simulink model "TCMSSystem"  (R2019b)
settings: configuration reference "ConfigSet_TCMSSystem_Reference" (kept outside this file)
model workspace (MAT data in the model file):
  Prm_TCMSSystem : Simulink.Parameter (value not decoded)
  SampleTime = 0.05
symbols that are objects in the model workspace (value not decoded): Prm_TCMSSystem
undefined symbols (not defined in the file): ADDIntervention, AK1Status, AK2Status, AKContactorStatus, AllDoorsClosed, AllLeftDoorsClosed, AllRightDoorsClosed, APS1Fault, APS1Isolated, APS1OutputVoltage, APS1Status, APS2Fault, APS2Isolated, APS2OutputVoltage, APS2Status, APSKAKContactor, ASCOEnd1, ASCOEnd2, ATBMode, ATCBypassMode, ATCStatusNotOK, ATOMode, ATPLowSpeedCutoutStatus, ATPMode, AuxCompressor, BatteryCurrent, BatteryIsolationContactor, BatteryTemperature, BatteryVoltage, BCG1Fault, BCG1Isolated, BCG1IsolationFailed, BCG1OutputCurrent, BCG1Status, BCG2Fault, BCG2Isolated, BCG2OutputCurrent, BCG2Status, BCGOutputVoltage, BECU1AxleLockedWheelSet1, BECU2AxleLockedWheelSet2, BECUFaulty, BECUMajorFault, BECUMinorFault, BECUStatus, BIC1Inside, BIC1Outside, BIC2Inside, BIC2Outside, Bogie, Bogie1WSPStatus, Bogie2WSPStatus, BogieFaulty, BogieIsolationStatus, BogieSupportedMass, BrakeCylinderPressureGauge, BrakeLoopCBTripped, BrakeLoopOpenTL, BrakeTrainLineStatus, BrakingDemand ... (+215)
libraries: TimersLib x257, simulink x137, LatchesLib x42, VectorOperationsLib x15, TestBenchLib x12, MathOperationsLib x2, FiltersLib x1
(part 12 of 16)

== system TCMSSystem/TCMSSystemPerVehicle/EnabledTCMSVehicle/TCMSTractionBraking/TractionBrakingControl/CabControlsExtract/CabActiveTrainControl ==
  In Bus Element6 : Inport  PortName=DisplayControl  Element=EnableTractionPowerLimit
  In Bus Element5 : Inport  PortName=DisplayControl  Element=EDBrakingPowerLimit
  In Bus Element7 : Inport  PortName=DisplayControl  Element=EnableEDBrakingPowerLimit
  In Bus Element8 : Inport  PortName=DisplayControl  Element=MaxTractionAccelerationTargetOverride
  In Bus Element : Inport  PortName=DisplayControl  Element=MaxBrakingDecelerationTargetOverride
  In Bus Element1 : Inport  PortName=DisplayControl  Element=EnableTractionTargetOverride
  In Bus Element2 : Inport  PortName=DisplayControl  Element=EnableBrakingTargetOverride
  In Bus Element4 : Inport  PortName=DisplayControl  Element=TractionPowerLimit
  TractionCommand : Inport  Port=2
  BrakingCommand : Inport  Port=3
  HoldingBrakeStatus : Inport  Port=4
  TCMSSpeedLimit : Inport  Port=5
  LimitActive : Inport  Port=6
  HTERequired : Inport  Port=7
  WashModeActive : Inport  Port=8
  ShuntModeActive : Inport  Port=9
  ATPLowSpeedCutoutModeActive : Inport  Port=10
  Action Port : ActionPort  ActionPortLabel=if(u1 > 0)
  Bus Creator : BusCreator  Inputs=19  OutDataTypeStr=Bus: BD_TCMSSystem_Wires_TBTrainWire  NonVirtualBus=on
  Constant : Constant  Value=0
  Constant1 : Constant  Value=0
  Out1 : Outport
  wires:
  Bus Creator/1 -> Out1/1
  In Bus Element4/1 -> Bus Creator/1  "TractionPowerLimit"
  In Bus Element5/1 -> Bus Creator/2  "EDBrakingPowerLimit"
  In Bus Element6/1 -> Bus Creator/3  "EnableTractionPowerLimit"
  In Bus Element8/1 -> Bus Creator/5  "MaxTractionAccelerationTargetOverride"
  In Bus Element7/1 -> Bus Creator/4  "EnableEDBrakingPowerLimit"
  In Bus Element/1 -> Bus Creator/6  "MaxBrakingDecelerationTargetOverride"
  In Bus Element1/1 -> Bus Creator/7  "EnableTractionTargetOverride"
  In Bus Element2/1 -> Bus Creator/8  "EnableBrakingTargetOverride"
  BrakingCommand/1 -> Bus Creator/10  "BrakingCommand"
  TractionCommand/1 -> Bus Creator/9  "TractionCommand"
  HoldingBrakeStatus/1 -> Bus Creator/11  "HoldingBrakeStatus"
  TCMSSpeedLimit/1 -> Bus Creator/12  "TCMSSpeedLimit"
  LimitActive/1 -> Bus Creator/13  "Overspeed"
  Constant/1 -> Bus Creator/14  "EstimatedMass"
  HTERequired/1 -> Bus Creator/15  "HTERequired"
  WashModeActive/1 -> Bus Creator/16  "WashModeActive"
  Constant1/1 -> Bus Creator/17  "TractionForce"
  ShuntModeActive/1 -> Bus Creator/18  "ShuntModeActive"
  ATPLowSpeedCutoutModeActive/1 -> Bus Creator/19  "ATPLowSpeedCutoutModeActive"

== system TCMSSystem/TCMSSystemPerVehicle/EnabledTCMSVehicle/TCMSTractionBraking/TractionBrakingControl/CabControlsExtract/CabInactiveNoTrainControl ==
  Action Port : ActionPort  ActionPortLabel=else
  Constant3 : Constant  Value=0  OutDataTypeStr=Bus: BD_TCMSSystem_Wires_TBTrainWire
  Out1 : Outport
  wires:
  Constant3/1 -> Out1/1

== system TCMSSystem/TCMSSystemPerVehicle/EnabledTCMSVehicle/TCMSTractionBraking/TractionBrakingControl/CabControlsExtract/Speed Limit Protection ==
  ElectricalIn : Inport
  CBTCIn : Inport  Port=2
  IOControls : Inport  Port=3
  In Bus Element7 : Inport  Port=4  PortName=DisplayControl
  In Bus Element : Inport  Port=4  PortName=DisplayControl  Element=ActivateWashing3Kmph
  In Bus Element1 : Inport  Port=4  PortName=DisplayControl  Element=ActivateWashing4Kmph
  In Bus Element2 : Inport  Port=4  PortName=DisplayControl  Element=ActivateWashing5Kmph
  In Bus Element3 : Inport  Port=4  PortName=DisplayControl  Element=ShuntModeMaxSpeed
  In Bus Element4 : Inport  Port=4  PortName=DisplayControl  Element=ATPLowModeMaxSpeed
  In Bus Element5 : Inport  Port=4  PortName=DisplayControl  Element=ATPLowModeActivated
  In Bus Element6 : Inport  Port=4  PortName=DisplayControl  Element=ShuntModeActivated
  PneumaticsSystem : Inport  Port=5
  PneumaticsTrainSum : Inport  Port=6
  TractionBrakingBogieData : Inport  Port=7
  0kphConditions : Subsystem
  10kphConditions : Subsystem
  25kphConditions : Subsystem
  40kphConditions : Subsystem
  45kphConditions : Subsystem
  50kphConditions : Subsystem
  Bus Selector : BusSelector  OutputSignals=Speedometer
  Bus Selector2 : BusSelector  OutputSignals=Bogie
  Constant : Constant  Value=0
  Constant1 : Constant  Value=40
  Constant2 : Constant  Value=25
  Constant3 : Constant  Value=45
  Constant4 : Constant  Value=50
  Constant5 : Constant  Value=10
  Constant6 : Constant  Value=3
  Constant7 : Constant  Value=4
  Constant8 : Constant  Value=5
  OR : Logic  Operator=OR  Inputs=3  AllPortsSameDT=off  OutDataTypeStr=boolean
  SetByATCLimits : Constant  Value=0
  Special Modes Case : Subsystem
  Switch{,1..10} (11 alike) : Switch  Criteria=u2 > Threshold
  kphTomps{1..11} (11 alike) : Gain  Gain=1/3.6
  SpecialModesOverspeed : Outport
  TCMSSpeedLimit : Outport  Port=2
  LimitActive : Outport  Port=3
  WashModeActive : Outport  Port=4
  wires:
  Constant/1 -> Switch/1
  Constant2/1 -> kphTomps1/1
  kphTomps1/1 -> Switch2/1
  0kphConditions/1(True) -> Special Modes Case/7(SpeedRestrict), Switch/2  "6 or more bogies isolated"
  25kphConditions/1(True) -> Switch2/2  "LimpHome or Forward Mode"
  ElectricalIn/1 -> 40kphConditions/1(ElectricalIn), 25kphConditions/3(ElectricalIn), Bus Selector/1
  Switch2/1 -> Switch5/3
  CBTCIn/1 -> 10kphConditions/2(CBTCIn), 0kphConditions/3(CBTCIn), Special Modes Case/1(CBTCIn), 25kphConditions/2(CBTCIn)
  Bus Selector/1 -> Special Modes Case/3(<Speedometer>)  "<Speedometer>"
  40kphConditions/1(True) -> Switch1/2  "4 or more bogies isolated"
  kphTomps2/1 -> Switch10/3
  SetByATCLimits/1 -> kphTomps2/1
  Switch1/1 -> Switch2/3
  Constant1/1 -> kphTomps3/1
  45kphConditions/1(True) -> Switch3/2  "3 or more bogies isolated"
  Switch3/1 -> Switch1/3
  Constant3/1 -> kphTomps4/1
  50kphConditions/1(True) -> Switch4/2  "2 or more bogies isolated"
  Switch4/1 -> Switch3/3
  Constant4/1 -> kphTomps5/1
  kphTomps3/1 -> Switch1/1
  kphTomps4/1 -> Switch3/1
  kphTomps5/1 -> Switch4/1
  10kphConditions/1(True) -> Switch5/2  "Reverse mode"
  Switch5/1 -> Switch6/3
  Constant5/1 -> kphTomps6/1
  kphTomps6/1 -> Switch5/1
  Switch/1 -> Special Modes Case/4(SpeedLimit), TCMSSpeedLimit/1
  PneumaticsTrainSum/1 -> 45kphConditions/1(PneumaticTrainSum), 10kphConditions/1(PneumaticsIn), 0kphConditions/1(PneumaticTrainSum), 40kphConditions/2(PneumaticTrainSum), 50kphConditions/2(PneumaticTrainSum)
  TractionBrakingBogieData/1 -> 50kphConditions/3(TractionBrakingBogieData), 40kphConditions/3(TractionBrakingBogieData)
  Switch7/1 -> Switch/3
  Switch8/1 -> Switch7/3
  Switch6/1 -> Switch8/3
  In Bus Element/1 -> OR/1, Switch7/2
  In Bus Element1/1 -> OR/2, Switch8/2
  In Bus Element2/1 -> OR/3, Switch6/2
  kphTomps7/1 -> Switch7/1
  Constant6/1 -> kphTomps7/1
  Constant7/1 -> kphTomps8/1
  kphTomps8/1 -> Switch8/1
  kphTomps9/1 -> Switch6/1
  Constant8/1 -> kphTomps9/1
  PneumaticsSystem/1 -> Bus Selector2/1
  Bus Selector2/1 -> 40kphConditions/4(<Bogie>), 50kphConditions/1(<Bogie>)  "<Bogie>"
  OR/1 -> WashModeActive/1, Special Modes Case/2(WashModeActive)  "WashModeActive"
  IOControls/1 -> 0kphConditions/2(IOControls), Special Modes Case/5(IOControls), 25kphConditions/1(IOControls), 10kphConditions/3(IOControls)
  Special Modes Case/1(SpecialModesOverspeed) -> SpecialModesOverspeed/1
  Special Modes Case/2(SpecialLimitActive) -> LimitActive/1
  Switch9/1 -> Switch4/3
  kphTomps10/1 -> Switch9/1
  In Bus Element3/1 -> kphTomps10/1
  Switch10/1 -> Switch9/3
  In Bus Element6/1 -> Switch9/2
  In Bus Element4/1 -> kphTomps11/1
  In Bus Element5/1 -> Switch10/2
  In Bus Element7/1 -> Special Modes Case/6(DisplayControl)
  kphTomps11/1 -> Switch10/1

== system TCMSSystem/TCMSSystemPerVehicle/EnabledTCMSVehicle/TCMSTractionBraking/TractionBrakingControl/CabControlsExtract/TractionBrakingRefCalc ==
  note: In wash mode, for example, for 3KMPH set point, traction will be cut at 3 kmph,
      | 50% FSB shall be applied at 4 KMPH, and FSB shall be applied at 5 KMPH.
      | This logic is extended for 4 and 5 KMPH set points.
  note: TractionCutoutFault
  DynamicsIn : Inport
  CBTCSignals : Inport  Port=2
  InputState : Inport  Port=3
  TractionCmd : Inport  Port=4
  In Bus Element26 : Inport  Port=5  PortName=Faults  Element=BECUPWRAndBRKCmdAtSameTime
  In Bus Element : Inport  Port=5  PortName=Faults  Element=TractionCutModeSelectorInATPATOUTO
  SpecialModesOverspeed : Inport  Port=6
  Abs : Abs
  Bus Selector : BusSelector  OutputSignals=TractionBrakeController,ModeSelector
  Bus Selector1 : BusSelector  OutputSignals=VehicleSpeed
  Bus Selector2 : BusSelector  OutputSignals=BrakingCommand,TractionForce
  Bus Selector4 : BusSelector  OutputSignals=HoldingBrakeStatus
  Compare To Constant : simulink/Logic and Bit Operations/Compare To Constant  relop===  const=0  OutDataTypeStr=boolean
  Compare To Constant1 : simulink/Logic and Bit Operations/Compare To Constant  relop===  const=4  OutDataTypeStr=boolean
  Compare To Constant2 : simulink/Logic and Bit Operations/Compare To Constant  relop===  const=5  OutDataTypeStr=boolean
  Compare To Constant4 : simulink/Logic and Bit Operations/Compare To Constant  relop===  const=1  OutDataTypeStr=boolean
  Compare To Constant5 : simulink/Logic and Bit Operations/Compare To Constant  relop===  const=2  OutDataTypeStr=boolean
  Constant : Constant  Value=0
  Constant1 : Constant  Value=100
  Constant2 : Constant  Value=0
  Constant3 : Constant  Value=50
  Constant4 : Constant  Value=100
  Detect Increase : simulink/Logic and Bit Operations/Detect Increase  vinit=0.0  OutDataTypeStr=boolean
  Detect Increase1 : simulink/Logic and Bit Operations/Detect Increase  vinit=0.0  OutDataTypeStr=boolean
  HBRelease : Subsystem
  HoldingBrake : Subsystem
  Logical Operator : Logic  Operator=OR  Inputs=3  AllPortsSameDT=off  OutDataTypeStr=boolean
  Logical Operator1 : Logic  Operator=OR  AllPortsSameDT=off  OutDataTypeStr=boolean
  Logical Operator2 : Logic  Operator=OR  AllPortsSameDT=off  OutDataTypeStr=boolean
  Logical Operator3 : Logic  AllPortsSameDT=off  OutDataTypeStr=boolean
  Max : MinMax  Function=max  Inputs=2
  SR Latch - Reset Priority : LatchesLib/SR Latch - Reset Priority  initial_condition=0
      settings: SourceProductName=Latches
  Saturation : Saturate  UpperLimit=120  LowerLimit=0
  Saturation1 : Saturate  UpperLimit=0  LowerLimit=-120
  Switch{,1..6} (7 alike) : Switch  Criteria=u2 > Threshold
  TBRefDemandFromCBTC : Subsystem
  TractionCommand : Outport
  BrakingCommand : Outport  Port=2
  HoldingBrakesStatus : Outport  Port=3
  wires:
  TBRefDemandFromCBTC/1(ATO/UTOModeActive) -> [ATOMode], Switch2/2, Switch1/2
  CBTCSignals/1 -> TBRefDemandFromCBTC/1(CBTC)
  TBRefDemandFromCBTC/2(RefTraction) -> Switch1/1
  Switch5/1 -> BrakingCommand/1
  InputState/1 -> Bus Selector/1
  TBRefDemandFromCBTC/3(RefBraking) -> Switch2/1
  Saturation/1 -> Switch1/3  "TractionCommand"
  Bus Selector/1 -> Saturation1/1, Saturation/1  "<TractionBrakeController>"
  Saturation1/1 -> Abs/1
  Abs/1 -> Switch2/3  "BrakingCommand"
  HoldingBrake/1(HoldingBrakeDemand) -> Max/2
  HoldingBrake/2(HoldingBrakeApplied) -> HoldingBrakesStatus/1  "HoldingBrakeApplied"
  DynamicsIn/1 -> Bus Selector1/1
  Bus Selector1/1 -> HoldingBrake/2(VehicleSpeed)  "<VehicleSpeed>"
  HBRelease/1(HBRelease) -> HoldingBrake/3(TCMSHoldingBrakeRelease)
  [NotImmobilise] -> HBRelease/2(NotImmobilise)
  [ATOMode] -> HBRelease/3(ATO/UTO)
  TBRefDemandFromCBTC/5(NotImmobilise) -> [NotImmobilise]
  TBRefDemandFromCBTC/4(NoSB) -> Switch3/2, Switch/2
  Switch2/1 -> Switch3/1
  Switch1/1 -> Switch/1
  Switch4/1 -> TractionCommand/1
  Constant1/1 -> Switch3/3
  Constant/1 -> Switch/3
  TractionCmd/1 -> Bus Selector4/1, Bus Selector2/1
  Switch3/1 -> Max/1
  Bus Selector4/1 -> HBRelease/4(HBStatus)  "<HoldingBrakeStatus>"
  Switch/1 -> Switch4/3
  Bus Selector/2 -> [ModeSelector]  "<ModeSelector>"
  [ModeSelector] -> Compare To Constant2/1, Compare To Constant1/1, Compare To Constant/1
  Compare To Constant/1 -> Detect Increase1/1, Logical Operator/1
  Compare To Constant1/1 -> Logical Operator/2
  Compare To Constant2/1 -> Logical Operator/3
  Logical Operator/1 -> Logical Operator3/1
  Constant2/1 -> Switch4/1
  In Bus Element/1 -> Logical Operator3/2
  Logical Operator1/1 -> Switch4/2
  In Bus Element26/1 -> Detect Increase/1
  Detect Increase/1 -> SR Latch - Reset Priority/1
  Constant4/1 -> Switch5/1
  Logical Operator3/1 -> Logical Operator1/2
  Detect Increase1/1 -> SR Latch - Reset Priority/2
  Max/1 -> Switch6/3
  SpecialModesOverspeed/1 -> Compare To Constant5/1, Compare To Constant4/1
  SR Latch - Reset Priority/1 -> Logical Operator2/1, Logical Operator1/1
  Compare To Constant4/1 -> Logical Operator2/2
  Logical Operator2/1 -> Switch5/2
  Compare To Constant5/1 -> Switch6/2
  Constant3/1 -> Switch6/1
  Switch6/1 -> Switch5/3
  Bus Selector2/2 -> HBRelease/1(TractionForceFB)  "<TractionForce>"
  Bus Selector2/1 -> HoldingBrake/1(BrakingCommand)  "<BrakingCommand>"

== system TCMSSystem/TCMSSystemPerVehicle/EnabledTCMSVehicle/TCMSTractionBraking/TractionBrakingControl/ForEachBogie/Subsystem ==
  note: Brake blending, EP compensates what ED cannot provide
  note: SH: This update was done in Nov24 because the brake icon on brake screen should not
      | glow for T car until the speed is less than 7 KMPH.
      | Total brake demand is calculated per unit, hence it is important to compare it with
      | the ED brake achieved per unit in order to calculate the EP demand (deficit). But at lower speed
      | when ED efforts are fading out, the brake demand is compared per vehicle and T cars are the first one to get the EP demand,
      | until there is still some ED brake efforts possible in DM/M cars.
      | This also improves the max and avg acceleration (ED+EP).
  EffortsAchievedPerUnit : Inport
  Speed : Inport  Port=2
  EffortsAchivedPerVehicle : Inport  Port=3
  Abs : Abs
  Bus Selector2 : BusSelector  OutputSignals=EDBrakingEffortAchieved
  Bus Selector3 : BusSelector  OutputSignals=EDBrakingEffortAchieved
  Bus Selector4 : BusSelector  OutputSignals=VehicleSpeed
  Switch1 : Switch  Criteria=u2 > Threshold  Threshold=1.75
  SelectEPBrakeDemand : Outport
  wires:
  Bus Selector3/1 -> Switch1/1  "<EDBrakingEffortAchieved>"
  Switch1/1 -> SelectEPBrakeDemand/1
  Bus Selector2/1 -> Switch1/3  "<EDBrakingEffortAchieved>"
  EffortsAchivedPerVehicle/1 -> Bus Selector2/1
  Bus Selector4/1 -> Abs/1  "<VehicleSpeed>"
  Abs/1 -> Switch1/2
  EffortsAchievedPerUnit/1 -> Bus Selector3/1
  Speed/1 -> Bus Selector4/1

== system TCMSSystem/TCMSSystemPerVehicle/EnabledTCMSVehicle/TCMSTractionBraking/TractionBrakingDisplay/BrakeScreen/For Each Subsystem ==
  In1 : Inport  Partition=on  PartitionDimension=1  PartitionWidth=1  PartitionOffset=0
  Bus Selector : BusSelector  OutputSignals=TCUSlideDetected,EDBrakeNotIsolated,TCUSlipDetected
  For Each : ForEach  DisableCoverage=on
  SlideDetected : Outport  ConcatenationDimension=1
  SlipDetected : Outport  Port=2  ConcatenationDimension=1
  EDBrakeAvailable : Outport  Port=3  ConcatenationDimension=1
  wires:
  In1/1 -> Bus Selector/1
  Bus Selector/1 -> SlideDetected/1  "<TCUSlideDetected>"
  Bus Selector/3 -> SlipDetected/1  "<TCUSlipDetected>"
  Bus Selector/2 -> EDBrakeAvailable/1  "<EDBrakeNotIsolated>"

== system TCMSSystem/TCMSSystemPerVehicle/EnabledTCMSVehicle/TCMSTractionBraking/TractionBrakingDisplay/OperatingandOtherScreen/CabUnitDisplay ==
  TCMSConfig : Inport
  ElectricalSignals : Inport  Port=2
  TractionUnitData : Inport  Port=3
  AND : Logic  AllPortsSameDT=off  OutDataTypeStr=boolean
  Bus Selector : BusSelector  OutputSignals=CabActive
  Bus Selector1 : BusSelector  OutputSignals=HasCab
  CabActiveUnitDisplay : Subsystem  TreatAsAtomicUnit=on
  CabInactiveNoDisplay : Subsystem  TreatAsAtomicUnit=on
  Data Type Conversion : DataTypeConversion  OutDataTypeStr=uint32
  If : If
  Merge : Merge
  CabUnitDisplay : Outport
  wires:
  Merge/1 -> CabUnitDisplay/1
  CabInactiveNoDisplay/1(Out1) -> Merge/2
  CabActiveUnitDisplay/1(Out1) -> Merge/1
  If/2 -> CabInactiveNoDisplay/Action
  If/1 -> CabActiveUnitDisplay/Action
  Data Type Conversion/1 -> If/1
  AND/1 -> Data Type Conversion/1
  Bus Selector/1 -> AND/2  "<CabActive>"
  Bus Selector1/1 -> AND/1  "<HasCab>"
  TCMSConfig/1 -> Bus Selector1/1
  ElectricalSignals/1 -> Bus Selector/1, CabActiveUnitDisplay/1(ElectricalSignals)
  TractionUnitData/1 -> CabActiveUnitDisplay/2(TractionUnitData)

== system TCMSSystem/TCMSSystemPerVehicle/EnabledTCMSVehicle/TCMSTractionBraking/TractionBrakingDisplay/PropulsionScreen/For Each Subsystem ==
  In1 : Inport  Partition=on  PartitionDimension=1  PartitionWidth=1  PartitionOffset=0
  In2 : Inport  Port=2  Partition=on  PartitionDimension=1  PartitionWidth=1  PartitionOffset=0
  Bus Selector : BusSelector  OutputSignals=EDBrakeNotIsolated
  Bus Selector1 : BusSelector  OutputSignals=WSPTractionCutout
  For Each : ForEach  DisableCoverage=on
  EDBrakeAvailable : Outport  ConcatenationDimension=1
  HeavyWheelSlipDetected : Outport  Port=2  ConcatenationDimension=1
  wires:
  In1/1 -> Bus Selector/1
  Bus Selector/1 -> EDBrakeAvailable/1  "<EDBrakeNotIsolated>"
  In2/1 -> Bus Selector1/1
  Bus Selector1/1 -> HeavyWheelSlipDetected/1  "<WSPTractionCutout>"

== system TCMSSystem/TCMSSystemPerVehicle/LimpHomeTCMSVehicle/TCMSTractionBraking/TractionBrakingControl/CabControlsExtract/CabActiveTrainControl ==
  In Bus Element6 : Inport  PortName=DisplayControl  Element=EnableTractionPowerLimit
  In Bus Element5 : Inport  PortName=DisplayControl  Element=EDBrakingPowerLimit
  In Bus Element7 : Inport  PortName=DisplayControl  Element=EnableEDBrakingPowerLimit
  In Bus Element8 : Inport  PortName=DisplayControl  Element=MaxTractionAccelerationTargetOverride
  In Bus Element : Inport  PortName=DisplayControl  Element=MaxBrakingDecelerationTargetOverride
  In Bus Element1 : Inport  PortName=DisplayControl  Element=EnableTractionTargetOverride
  In Bus Element2 : Inport  PortName=DisplayControl  Element=EnableBrakingTargetOverride
  In Bus Element4 : Inport  PortName=DisplayControl  Element=TractionPowerLimit
  TractionCommand : Inport  Port=2
  BrakingCommand : Inport  Port=3
  HoldingBrakeStatus : Inport  Port=4
  TCMSSpeedLimit : Inport  Port=5
  LimitActive : Inport  Port=6
  Action Port : ActionPort  ActionPortLabel=if(u1 > 0)
  Bus Creator : BusCreator  Inputs=19  OutDataTypeStr=Bus: BD_TCMSSystem_Wires_TBTrainWire  NonVirtualBus=on
  Constant{,1..5} (6 alike) : Constant  Value=0
  Out1 : Outport
  wires:
  Bus Creator/1 -> Out1/1
  In Bus Element4/1 -> Bus Creator/1  "TractionPowerLimit"
  In Bus Element5/1 -> Bus Creator/2  "EDBrakingPowerLimit"
  In Bus Element6/1 -> Bus Creator/3  "EnableTractionPowerLimit"
  In Bus Element8/1 -> Bus Creator/5  "MaxTractionAccelerationTargetOverride"
  In Bus Element7/1 -> Bus Creator/4  "EnableEDBrakingPowerLimit"
  In Bus Element/1 -> Bus Creator/6  "MaxBrakingDecelerationTargetOverride"
  In Bus Element1/1 -> Bus Creator/7  "EnableTractionTargetOverride"
  In Bus Element2/1 -> Bus Creator/8  "EnableBrakingTargetOverride"
  BrakingCommand/1 -> Bus Creator/10  "BrakingCommand"
  TractionCommand/1 -> Bus Creator/9  "TractionCommand"
  HoldingBrakeStatus/1 -> Bus Creator/11  "HoldingBrakeStatus"
  TCMSSpeedLimit/1 -> Bus Creator/12  "TCMSSpeedLimit"
  LimitActive/1 -> Bus Creator/13  "Overspeed"
  Constant/1 -> Bus Creator/14  "EstimatedMass"
  Constant1/1 -> Bus Creator/15  "HTERequired"
  Constant2/1 -> Bus Creator/16  "WashModeActive"
  Constant3/1 -> Bus Creator/17  "TractionForce"
  Constant4/1 -> Bus Creator/18  "ShuntModeActive"
  Constant5/1 -> Bus Creator/19  "ATPLowSpeedCutoutModeActive"

== system TCMSSystem/TCMSSystemPerVehicle/LimpHomeTCMSVehicle/TCMSTractionBraking/TractionBrakingControl/CabControlsExtract/CabInactiveNoTrainControl ==
  Action Port : ActionPort  ActionPortLabel=else
  Constant3 : Constant  Value=0  OutDataTypeStr=Bus: BD_TCMSSystem_Wires_TBTrainWire
  Out1 : Outport
  wires:
  Constant3/1 -> Out1/1

== system TCMSSystem/TCMSSystemPerVehicle/LimpHomeTCMSVehicle/TCMSTractionBraking/TractionBrakingControl/CabControlsExtract/Speed Limit Protection ==
  note: This speed limit shall be displayed on HMI header.
  ElectricalIn : Inport
  PneumaticTrainSum : Inport  Port=2
  CBTCIn : Inport  Port=3
  IOControl : Inport  Port=4
  0kphConditions : Subsystem
  10kphConditions : Subsystem
  Bus Selector : BusSelector  OutputSignals=Speedometer
  Constant : Constant  Value=0
  Constant2 : Constant  Value=25
  Constant5 : Constant  Value=10
  Data Type Conversion : DataTypeConversion
  Relational Operator : RelationalOperator  OutDataTypeStr=boolean  RndMeth=Simplest
  Switch : Switch  Criteria=u2 > Threshold
  Switch5 : Switch  Criteria=u2 > Threshold
  TCMSDisplaySpeedLim : Subsystem
  kphTomps1 : Gain  Gain=1/3.6
  kphTomps6 : Gain  Gain=1/3.6
  TCMSSpeedLimit : Outport
  LimitActive : Outport  Port=2
  wires:
  Constant/1 -> Switch/1
  Constant2/1 -> kphTomps1/1
  0kphConditions/1(True) -> Switch/2
  Switch/1 -> Relational Operator/2  "TCMS Speed Limit"
  ElectricalIn/1 -> Bus Selector/1
  kphTomps1/1 -> Switch5/3
  CBTCIn/1 -> 10kphConditions/1(CBTCIn)
  Relational Operator/1 -> Data Type Conversion/1
  Bus Selector/1 -> Relational Operator/1  "<Speedometer>"
  Data Type Conversion/1 -> LimitActive/1
  10kphConditions/1(True) -> Switch5/2
  Switch5/1 -> Switch/3
  Constant5/1 -> kphTomps6/1
  kphTomps6/1 -> Switch5/1
  IOControl/1 -> TCMSDisplaySpeedLim/1(IOControl)
  TCMSDisplaySpeedLim/1(TCMSSpeedLimit) -> TCMSSpeedLimit/1
  PneumaticTrainSum/1 -> 0kphConditions/1(PneumaticTrainSum)

== system TCMSSystem/TCMSSystemPerVehicle/LimpHomeTCMSVehicle/TCMSTractionBraking/TractionBrakingControl/CabControlsExtract/TractionBrakingRefCalc ==
  ElectricalSignals : Inport
  In4 : Inport  Port=2
  Bus Selector1 : BusSelector  OutputSignals=ZeroSpeed
  Bus Selector2 : BusSelector  OutputSignals=TractionCommand
  Bus Selector4 : BusSelector  OutputSignals=MotorTrainLine,BrakeTrainLine,FSB1Line,FSB2Line
  Constant1 : Constant  Value=0
  Constant2 : Constant  Value=100
  Constant3 : Constant  Value=70
  Constant4 : Constant  Value=0
  HBRelease : Subsystem
  HoldingBrake : Subsystem
  Logical Operator2 : Logic  Operator=NAND  Inputs=3  AllPortsSameDT=off  OutDataTypeStr=boolean
  Max : MinMax  Function=max  Inputs=2
  Switch4 : Switch  Criteria=u2 > Threshold
  Switch5 : Switch  Criteria=u2 > Threshold
  TractionCommand : Outport
  BrakingCommand : Outport  Port=2
  HoldingBrakesStatus : Outport  Port=3
  wires:
  Max/1 -> BrakingCommand/1
  HoldingBrake/1(HoldingBrakeDemand) -> Max/2
  HoldingBrake/2(HoldingBrakeApplied) -> HoldingBrakesStatus/1  "HoldingBrakeApplied"
  ElectricalSignals/1 -> [ElectricalIn], Bus Selector1/1
  Bus Selector1/1 -> HoldingBrake/2(ZeroSpeed)  "<ZeroSpeed>"
  HBRelease/1(HBRelease) -> HoldingBrake/3(TCMSHoldingBrakeRelease)
  Constant4/1 -> Switch5/3
  Switch4/1 -> TractionCommand/1
  In4/1 -> Bus Selector2/1
  Bus Selector2/1 -> HBRelease/1(TractionRef), HoldingBrake/1(TractionCmd)  "<TractionCommand>"
  Switch5/1 -> Max/1
  Constant1/1 -> Switch4/3
  Constant2/1 -> Switch4/1
  Logical Operator2/1 -> Switch5/2
  Constant3/1 -> Switch5/1
  [ElectricalIn] -> Bus Selector4/1
  Bus Selector4/3 -> Logical Operator2/2  "<FSB1Line>"
  Bus Selector4/4 -> Logical Operator2/3  "<FSB2Line>"
  Bus Selector4/2 -> Logical Operator2/1  "<BrakeTrainLine>"
  Bus Selector4/1 -> Switch4/2  "<MotorTrainLine>"

== system TCMSSystem/TCMSSystemPerVehicle/EnabledTCMSVehicle/OutputsPacking/TCMSDisplayOutputs/TCMSMessageEvents/BrakeSystemFaults/Associated TCMS Fault ID1 ==
  State : Inport
  Bus Creator1 : BusCreator  Inputs=2  OutDataTypeStr=Bus: BD_TCMSSystem_Out_Vehicle_Display_Message  NonVirtualBus=on
  Constant : Constant  Value=MessageID
  Data Type Conversion : DataTypeConversion
  Message : Outport  VectorParamsAs1DForOutWhenUnconnected=off
  wires:
  Bus Creator1/1 -> Message/1
  State/1 -> Data Type Conversion/1
  Constant/1 -> Bus Creator1/1  "MessageID"
  Data Type Conversion/1 -> Bus Creator1/2  "MessageStatus"

== system TCMSSystem/TCMSSystemPerVehicle/EnabledTCMSVehicle/OutputsPacking/TCMSDisplayOutputs/TCMSMessageEvents/BrakeSystemFaults/Associated TCMS Fault ID10 ==
  State : Inport
  Bus Creator1 : BusCreator  Inputs=2  OutDataTypeStr=Bus: BD_TCMSSystem_Out_Vehicle_Display_Message  NonVirtualBus=on
  Constant : Constant  Value=MessageID
  Data Type Conversion : DataTypeConversion
  Message : Outport  VectorParamsAs1DForOutWhenUnconnected=off
  wires:
  Bus Creator1/1 -> Message/1
  State/1 -> Data Type Conversion/1
  Constant/1 -> Bus Creator1/1  "MessageID"
  Data Type Conversion/1 -> Bus Creator1/2  "MessageStatus"

== system TCMSSystem/TCMSSystemPerVehicle/EnabledTCMSVehicle/OutputsPacking/TCMSDisplayOutputs/TCMSMessageEvents/BrakeSystemFaults/Associated TCMS Fault ID11 ==
  State : Inport
  Bus Creator1 : BusCreator  Inputs=2  OutDataTypeStr=Bus: BD_TCMSSystem_Out_Vehicle_Display_Message  NonVirtualBus=on
  Constant : Constant  Value=MessageID
  Data Type Conversion : DataTypeConversion
  Message : Outport  VectorParamsAs1DForOutWhenUnconnected=off
  wires:
  Data Type Conversion/1 -> Bus Creator1/2  "MessageStatus"
  Constant/1 -> Bus Creator1/1  "MessageID"
  State/1 -> Data Type Conversion/1
  Bus Creator1/1 -> Message/1

== system TCMSSystem/TCMSSystemPerVehicle/EnabledTCMSVehicle/OutputsPacking/TCMSDisplayOutputs/TCMSMessageEvents/BrakeSystemFaults/Associated TCMS Fault ID12 ==
  State : Inport
  Bus Creator1 : BusCreator  Inputs=2  OutDataTypeStr=Bus: BD_TCMSSystem_Out_Vehicle_Display_Message  NonVirtualBus=on
  Constant : Constant  Value=MessageID
  Data Type Conversion : DataTypeConversion
  Message : Outport  VectorParamsAs1DForOutWhenUnconnected=off
  wires:
  Data Type Conversion/1 -> Bus Creator1/2  "MessageStatus"
  Constant/1 -> Bus Creator1/1  "MessageID"
  State/1 -> Data Type Conversion/1
  Bus Creator1/1 -> Message/1

== system TCMSSystem/TCMSSystemPerVehicle/EnabledTCMSVehicle/OutputsPacking/TCMSDisplayOutputs/TCMSMessageEvents/BrakeSystemFaults/Associated TCMS Fault ID13 ==
  State : Inport
  Bus Creator1 : BusCreator  Inputs=2  OutDataTypeStr=Bus: BD_TCMSSystem_Out_Vehicle_Display_Message  NonVirtualBus=on
  Constant : Constant  Value=MessageID
  Data Type Conversion : DataTypeConversion
  Message : Outport  VectorParamsAs1DForOutWhenUnconnected=off
  wires:
  Bus Creator1/1 -> Message/1
  State/1 -> Data Type Conversion/1
  Constant/1 -> Bus Creator1/1  "MessageID"
  Data Type Conversion/1 -> Bus Creator1/2  "MessageStatus"

== system TCMSSystem/TCMSSystemPerVehicle/EnabledTCMSVehicle/OutputsPacking/TCMSDisplayOutputs/TCMSMessageEvents/BrakeSystemFaults/Associated TCMS Fault ID14 ==
  State : Inport
  Bus Creator1 : BusCreator  Inputs=2  OutDataTypeStr=Bus: BD_TCMSSystem_Out_Vehicle_Display_Message  NonVirtualBus=on
  Constant : Constant  Value=MessageID
  Data Type Conversion : DataTypeConversion
  Message : Outport  VectorParamsAs1DForOutWhenUnconnected=off
  wires:
  Bus Creator1/1 -> Message/1
  State/1 -> Data Type Conversion/1
  Constant/1 -> Bus Creator1/1  "MessageID"
  Data Type Conversion/1 -> Bus Creator1/2  "MessageStatus"

== system TCMSSystem/TCMSSystemPerVehicle/EnabledTCMSVehicle/OutputsPacking/TCMSDisplayOutputs/TCMSMessageEvents/BrakeSystemFaults/Associated TCMS Fault ID15 ==
  State : Inport
  Bus Creator1 : BusCreator  Inputs=2  OutDataTypeStr=Bus: BD_TCMSSystem_Out_Vehicle_Display_Message  NonVirtualBus=on
  Constant : Constant  Value=MessageID
  Data Type Conversion : DataTypeConversion
  Message : Outport  VectorParamsAs1DForOutWhenUnconnected=off
  wires:
  Bus Creator1/1 -> Message/1
  State/1 -> Data Type Conversion/1
  Constant/1 -> Bus Creator1/1  "MessageID"
  Data Type Conversion/1 -> Bus Creator1/2  "MessageStatus"

== system TCMSSystem/TCMSSystemPerVehicle/EnabledTCMSVehicle/OutputsPacking/TCMSDisplayOutputs/TCMSMessageEvents/BrakeSystemFaults/Associated TCMS Fault ID16 ==
  State : Inport
  Bus Creator1 : BusCreator  Inputs=2  OutDataTypeStr=Bus: BD_TCMSSystem_Out_Vehicle_Display_Message  NonVirtualBus=on
  Constant : Constant  Value=MessageID
  Data Type Conversion : DataTypeConversion
  Message : Outport  VectorParamsAs1DForOutWhenUnconnected=off
  wires:
  Data Type Conversion/1 -> Bus Creator1/2  "MessageStatus"
  Constant/1 -> Bus Creator1/1  "MessageID"
  State/1 -> Data Type Conversion/1
  Bus Creator1/1 -> Message/1

== system TCMSSystem/TCMSSystemPerVehicle/EnabledTCMSVehicle/OutputsPacking/TCMSDisplayOutputs/TCMSMessageEvents/BrakeSystemFaults/Associated TCMS Fault ID2 ==
  State : Inport
  Bus Creator1 : BusCreator  Inputs=2  OutDataTypeStr=Bus: BD_TCMSSystem_Out_Vehicle_Display_Message  NonVirtualBus=on
  Constant : Constant  Value=MessageID
  Data Type Conversion : DataTypeConversion
  Message : Outport  VectorParamsAs1DForOutWhenUnconnected=off
  wires:
  Data Type Conversion/1 -> Bus Creator1/2  "MessageStatus"
  Constant/1 -> Bus Creator1/1  "MessageID"
  State/1 -> Data Type Conversion/1
  Bus Creator1/1 -> Message/1

== system TCMSSystem/TCMSSystemPerVehicle/EnabledTCMSVehicle/OutputsPacking/TCMSDisplayOutputs/TCMSMessageEvents/BrakeSystemFaults/Associated TCMS Fault ID3 ==
  State : Inport
  Bus Creator1 : BusCreator  Inputs=2  OutDataTypeStr=Bus: BD_TCMSSystem_Out_Vehicle_Display_Message  NonVirtualBus=on
  Constant : Constant  Value=MessageID
  Data Type Conversion : DataTypeConversion
  Message : Outport  VectorParamsAs1DForOutWhenUnconnected=off
  wires:
  Bus Creator1/1 -> Message/1
  State/1 -> Data Type Conversion/1
  Constant/1 -> Bus Creator1/1  "MessageID"
  Data Type Conversion/1 -> Bus Creator1/2  "MessageStatus"

== system TCMSSystem/TCMSSystemPerVehicle/EnabledTCMSVehicle/OutputsPacking/TCMSDisplayOutputs/TCMSMessageEvents/BrakeSystemFaults/Associated TCMS Fault ID4 ==
  State : Inport
  Bus Creator1 : BusCreator  Inputs=2  OutDataTypeStr=Bus: BD_TCMSSystem_Out_Vehicle_Display_Message  NonVirtualBus=on
  Constant : Constant  Value=MessageID
  Data Type Conversion : DataTypeConversion
  Message : Outport  VectorParamsAs1DForOutWhenUnconnected=off
  wires:
  Bus Creator1/1 -> Message/1
  State/1 -> Data Type Conversion/1
  Constant/1 -> Bus Creator1/1  "MessageID"
  Data Type Conversion/1 -> Bus Creator1/2  "MessageStatus"

== system TCMSSystem/TCMSSystemPerVehicle/EnabledTCMSVehicle/OutputsPacking/TCMSDisplayOutputs/TCMSMessageEvents/BrakeSystemFaults/Associated TCMS Fault ID5 ==
  State : Inport
  Bus Creator1 : BusCreator  Inputs=2  OutDataTypeStr=Bus: BD_TCMSSystem_Out_Vehicle_Display_Message  NonVirtualBus=on
  Constant : Constant  Value=MessageID
  Data Type Conversion : DataTypeConversion
  Message : Outport  VectorParamsAs1DForOutWhenUnconnected=off
  wires:
  Data Type Conversion/1 -> Bus Creator1/2  "MessageStatus"
  Constant/1 -> Bus Creator1/1  "MessageID"
  State/1 -> Data Type Conversion/1
  Bus Creator1/1 -> Message/1

== system TCMSSystem/TCMSSystemPerVehicle/EnabledTCMSVehicle/OutputsPacking/TCMSDisplayOutputs/TCMSMessageEvents/BrakeSystemFaults/Associated TCMS Fault ID6 ==
  State : Inport
  Bus Creator1 : BusCreator  Inputs=2  OutDataTypeStr=Bus: BD_TCMSSystem_Out_Vehicle_Display_Message  NonVirtualBus=on
  Constant : Constant  Value=MessageID
  Data Type Conversion : DataTypeConversion
  Message : Outport  VectorParamsAs1DForOutWhenUnconnected=off
  wires:
  Bus Creator1/1 -> Message/1
  State/1 -> Data Type Conversion/1
  Constant/1 -> Bus Creator1/1  "MessageID"
  Data Type Conversion/1 -> Bus Creator1/2  "MessageStatus"

== system TCMSSystem/TCMSSystemPerVehicle/EnabledTCMSVehicle/OutputsPacking/TCMSDisplayOutputs/TCMSMessageEvents/BrakeSystemFaults/Associated TCMS Fault ID7 ==
  State : Inport
  Bus Creator1 : BusCreator  Inputs=2  OutDataTypeStr=Bus: BD_TCMSSystem_Out_Vehicle_Display_Message  NonVirtualBus=on
  Constant : Constant  Value=MessageID
  Data Type Conversion : DataTypeConversion
  Message : Outport  VectorParamsAs1DForOutWhenUnconnected=off
  wires:
  Data Type Conversion/1 -> Bus Creator1/2  "MessageStatus"
  Constant/1 -> Bus Creator1/1  "MessageID"
  State/1 -> Data Type Conversion/1
  Bus Creator1/1 -> Message/1

== system TCMSSystem/TCMSSystemPerVehicle/EnabledTCMSVehicle/OutputsPacking/TCMSDisplayOutputs/TCMSMessageEvents/BrakeSystemFaults/Associated TCMS Fault ID8 ==
  State : Inport
  Bus Creator1 : BusCreator  Inputs=2  OutDataTypeStr=Bus: BD_TCMSSystem_Out_Vehicle_Display_Message  NonVirtualBus=on
  Constant : Constant  Value=MessageID
  Data Type Conversion : DataTypeConversion
  Message : Outport  VectorParamsAs1DForOutWhenUnconnected=off
  wires:
  Bus Creator1/1 -> Message/1
  State/1 -> Data Type Conversion/1
  Constant/1 -> Bus Creator1/1  "MessageID"
  Data Type Conversion/1 -> Bus Creator1/2  "MessageStatus"

== system TCMSSystem/TCMSSystemPerVehicle/EnabledTCMSVehicle/OutputsPacking/TCMSDisplayOutputs/TCMSMessageEvents/BrakeSystemFaults/Associated TCMS Fault ID80 ==
  State : Inport
  Bus Creator1 : BusCreator  Inputs=2  OutDataTypeStr=Bus: BD_TCMSSystem_Out_Vehicle_Display_Message  NonVirtualBus=on
  Constant : Constant  Value=MessageID
  Data Type Conversion : DataTypeConversion
  Message : Outport  VectorParamsAs1DForOutWhenUnconnected=off
  wires:
  Data Type Conversion/1 -> Bus Creator1/2  "MessageStatus"
  Constant/1 -> Bus Creator1/1  "MessageID"
  State/1 -> Data Type Conversion/1
  Bus Creator1/1 -> Message/1

== system TCMSSystem/TCMSSystemPerVehicle/EnabledTCMSVehicle/OutputsPacking/TCMSDisplayOutputs/TCMSMessageEvents/BrakeSystemFaults/Associated TCMS Fault ID81 ==
  State : Inport
  Bus Creator1 : BusCreator  Inputs=2  OutDataTypeStr=Bus: BD_TCMSSystem_Out_Vehicle_Display_Message  NonVirtualBus=on
  Constant : Constant  Value=MessageID
  Data Type Conversion : DataTypeConversion
  Message : Outport  VectorParamsAs1DForOutWhenUnconnected=off
  wires:
  Data Type Conversion/1 -> Bus Creator1/2  "MessageStatus"
  Constant/1 -> Bus Creator1/1  "MessageID"
  State/1 -> Data Type Conversion/1
  Bus Creator1/1 -> Message/1

== system TCMSSystem/TCMSSystemPerVehicle/EnabledTCMSVehicle/OutputsPacking/TCMSDisplayOutputs/TCMSMessageEvents/BrakeSystemFaults/Associated TCMS Fault ID82 ==
  State : Inport
  Bus Creator1 : BusCreator  Inputs=2  OutDataTypeStr=Bus: BD_TCMSSystem_Out_Vehicle_Display_Message  NonVirtualBus=on
  Constant : Constant  Value=MessageID
  Data Type Conversion : DataTypeConversion
  Message : Outport  VectorParamsAs1DForOutWhenUnconnected=off
  wires:
  Bus Creator1/1 -> Message/1
  State/1 -> Data Type Conversion/1
  Constant/1 -> Bus Creator1/1  "MessageID"
  Data Type Conversion/1 -> Bus Creator1/2  "MessageStatus"

== system TCMSSystem/TCMSSystemPerVehicle/EnabledTCMSVehicle/OutputsPacking/TCMSDisplayOutputs/TCMSMessageEvents/BrakeSystemFaults/Associated TCMS Fault ID83 ==
  State : Inport
  Bus Creator1 : BusCreator  Inputs=2  OutDataTypeStr=Bus: BD_TCMSSystem_Out_Vehicle_Display_Message  NonVirtualBus=on
  Constant : Constant  Value=MessageID
  Data Type Conversion : DataTypeConversion
  Message : Outport  VectorParamsAs1DForOutWhenUnconnected=off
  wires:
  Data Type Conversion/1 -> Bus Creator1/2  "MessageStatus"
  Constant/1 -> Bus Creator1/1  "MessageID"
  State/1 -> Data Type Conversion/1
  Bus Creator1/1 -> Message/1

== system TCMSSystem/TCMSSystemPerVehicle/EnabledTCMSVehicle/OutputsPacking/TCMSDisplayOutputs/TCMSMessageEvents/BrakeSystemFaults/Associated TCMS Fault ID84 ==
  State : Inport
  Bus Creator1 : BusCreator  Inputs=2  OutDataTypeStr=Bus: BD_TCMSSystem_Out_Vehicle_Display_Message  NonVirtualBus=on
  Constant : Constant  Value=MessageID
  Data Type Conversion : DataTypeConversion
  Message : Outport  VectorParamsAs1DForOutWhenUnconnected=off
  wires:
  Data Type Conversion/1 -> Bus Creator1/2  "MessageStatus"
  Constant/1 -> Bus Creator1/1  "MessageID"
  State/1 -> Data Type Conversion/1
  Bus Creator1/1 -> Message/1

== system TCMSSystem/TCMSSystemPerVehicle/EnabledTCMSVehicle/OutputsPacking/TCMSDisplayOutputs/TCMSMessageEvents/BrakeSystemFaults/Associated TCMS Fault ID85 ==
  State : Inport
  Bus Creator1 : BusCreator  Inputs=2  OutDataTypeStr=Bus: BD_TCMSSystem_Out_Vehicle_Display_Message  NonVirtualBus=on
  Constant : Constant  Value=MessageID
  Data Type Conversion : DataTypeConversion
  Message : Outport  VectorParamsAs1DForOutWhenUnconnected=off
  wires:
  Bus Creator1/1 -> Message/1
  State/1 -> Data Type Conversion/1
  Constant/1 -> Bus Creator1/1  "MessageID"
  Data Type Conversion/1 -> Bus Creator1/2  "MessageStatus"

== system TCMSSystem/TCMSSystemPerVehicle/EnabledTCMSVehicle/OutputsPacking/TCMSDisplayOutputs/TCMSMessageEvents/BrakeSystemFaults/Associated TCMS Fault ID86 ==
  State : Inport
  Bus Creator1 : BusCreator  Inputs=2  OutDataTypeStr=Bus: BD_TCMSSystem_Out_Vehicle_Display_Message  NonVirtualBus=on
  Constant : Constant  Value=MessageID
  Data Type Conversion : DataTypeConversion
  Message : Outport  VectorParamsAs1DForOutWhenUnconnected=off
  wires:
  Data Type Conversion/1 -> Bus Creator1/2  "MessageStatus"
  Constant/1 -> Bus Creator1/1  "MessageID"
  State/1 -> Data Type Conversion/1
  Bus Creator1/1 -> Message/1

== system TCMSSystem/TCMSSystemPerVehicle/EnabledTCMSVehicle/OutputsPacking/TCMSDisplayOutputs/TCMSMessageEvents/BrakeSystemFaults/Associated TCMS Fault ID87 ==
  State : Inport
  Bus Creator1 : BusCreator  Inputs=2  OutDataTypeStr=Bus: BD_TCMSSystem_Out_Vehicle_Display_Message  NonVirtualBus=on
  Constant : Constant  Value=MessageID
  Data Type Conversion : DataTypeConversion
  Message : Outport  VectorParamsAs1DForOutWhenUnconnected=off
  wires:
  Bus Creator1/1 -> Message/1
  State/1 -> Data Type Conversion/1
  Constant/1 -> Bus Creator1/1  "MessageID"
  Data Type Conversion/1 -> Bus Creator1/2  "MessageStatus"

== system TCMSSystem/TCMSSystemPerVehicle/EnabledTCMSVehicle/OutputsPacking/TCMSDisplayOutputs/TCMSMessageEvents/BrakeSystemFaults/Associated TCMS Fault ID88 ==
  State : Inport
  Bus Creator1 : BusCreator  Inputs=2  OutDataTypeStr=Bus: BD_TCMSSystem_Out_Vehicle_Display_Message  NonVirtualBus=on
  Constant : Constant  Value=MessageID
  Data Type Conversion : DataTypeConversion
  Message : Outport  VectorParamsAs1DForOutWhenUnconnected=off
  wires:
  Data Type Conversion/1 -> Bus Creator1/2  "MessageStatus"
  Constant/1 -> Bus Creator1/1  "MessageID"
  State/1 -> Data Type Conversion/1
  Bus Creator1/1 -> Message/1

== system TCMSSystem/TCMSSystemPerVehicle/EnabledTCMSVehicle/OutputsPacking/TCMSDisplayOutputs/TCMSMessageEvents/BrakeSystemFaults/Associated TCMS Fault ID9 ==
  State : Inport
  Bus Creator1 : BusCreator  Inputs=2  OutDataTypeStr=Bus: BD_TCMSSystem_Out_Vehicle_Display_Message  NonVirtualBus=on
  Constant : Constant  Value=MessageID
  Data Type Conversion : DataTypeConversion
  Message : Outport  VectorParamsAs1DForOutWhenUnconnected=off
  wires:
  Data Type Conversion/1 -> Bus Creator1/2  "MessageStatus"
  Constant/1 -> Bus Creator1/1  "MessageID"
  State/1 -> Data Type Conversion/1
  Bus Creator1/1 -> Message/1

== system TCMSSystem/TCMSSystemPerVehicle/EnabledTCMSVehicle/OutputsPacking/TCMSDisplayOutputs/TCMSMessageEvents/DoorSystemFaults/Associated TCMS Fault ID1 ==
  State : Inport
  Bus Creator1 : BusCreator  Inputs=2  OutDataTypeStr=Bus: BD_TCMSSystem_Out_Vehicle_Display_Message  NonVirtualBus=on
  Constant : Constant  Value=MessageID
  Data Type Conversion : DataTypeConversion
  Message : Outport  VectorParamsAs1DForOutWhenUnconnected=off
  wires:
  Bus Creator1/1 -> Message/1
  State/1 -> Data Type Conversion/1
  Constant/1 -> Bus Creator1/1  "MessageID"
  Data Type Conversion/1 -> Bus Creator1/2  "MessageStatus"

== system TCMSSystem/TCMSSystemPerVehicle/EnabledTCMSVehicle/OutputsPacking/TCMSDisplayOutputs/TCMSMessageEvents/DoorSystemFaults/Associated TCMS Fault ID10 ==
  State : Inport
  Bus Creator1 : BusCreator  Inputs=2  OutDataTypeStr=Bus: BD_TCMSSystem_Out_Vehicle_Display_Message  NonVirtualBus=on
  Constant : Constant  Value=MessageID
  Data Type Conversion : DataTypeConversion
  Message : Outport  VectorParamsAs1DForOutWhenUnconnected=off
  wires:
  Data Type Conversion/1 -> Bus Creator1/2  "MessageStatus"
  Constant/1 -> Bus Creator1/1  "MessageID"
  State/1 -> Data Type Conversion/1
  Bus Creator1/1 -> Message/1

== system TCMSSystem/TCMSSystemPerVehicle/EnabledTCMSVehicle/OutputsPacking/TCMSDisplayOutputs/TCMSMessageEvents/DoorSystemFaults/Associated TCMS Fault ID109 ==
  State : Inport
  Bus Creator1 : BusCreator  Inputs=2  OutDataTypeStr=Bus: BD_TCMSSystem_Out_Vehicle_Display_Message  NonVirtualBus=on
  Constant : Constant  Value=MessageID
  Data Type Conversion : DataTypeConversion
  Message : Outport  VectorParamsAs1DForOutWhenUnconnected=off
  wires:
  Data Type Conversion/1 -> Bus Creator1/2  "MessageStatus"
  Constant/1 -> Bus Creator1/1  "MessageID"
  State/1 -> Data Type Conversion/1
  Bus Creator1/1 -> Message/1

== system TCMSSystem/TCMSSystemPerVehicle/EnabledTCMSVehicle/OutputsPacking/TCMSDisplayOutputs/TCMSMessageEvents/DoorSystemFaults/Associated TCMS Fault ID11 ==
  State : Inport
  Bus Creator1 : BusCreator  Inputs=2  OutDataTypeStr=Bus: BD_TCMSSystem_Out_Vehicle_Display_Message  NonVirtualBus=on
  Constant : Constant  Value=MessageID
  Data Type Conversion : DataTypeConversion
  Message : Outport  VectorParamsAs1DForOutWhenUnconnected=off
  wires:
  Bus Creator1/1 -> Message/1
  State/1 -> Data Type Conversion/1
  Constant/1 -> Bus Creator1/1  "MessageID"
  Data Type Conversion/1 -> Bus Creator1/2  "MessageStatus"

== system TCMSSystem/TCMSSystemPerVehicle/EnabledTCMSVehicle/OutputsPacking/TCMSDisplayOutputs/TCMSMessageEvents/DoorSystemFaults/Associated TCMS Fault ID110 ==
  State : Inport
  Bus Creator1 : BusCreator  Inputs=2  OutDataTypeStr=Bus: BD_TCMSSystem_Out_Vehicle_Display_Message  NonVirtualBus=on
  Constant : Constant  Value=MessageID
  Data Type Conversion : DataTypeConversion
  Message : Outport  VectorParamsAs1DForOutWhenUnconnected=off
  wires:
  Data Type Conversion/1 -> Bus Creator1/2  "MessageStatus"
  Constant/1 -> Bus Creator1/1  "MessageID"
  State/1 -> Data Type Conversion/1
  Bus Creator1/1 -> Message/1

== system TCMSSystem/TCMSSystemPerVehicle/EnabledTCMSVehicle/OutputsPacking/TCMSDisplayOutputs/TCMSMessageEvents/DoorSystemFaults/Associated TCMS Fault ID111 ==
  State : Inport
  Bus Creator1 : BusCreator  Inputs=2  OutDataTypeStr=Bus: BD_TCMSSystem_Out_Vehicle_Display_Message  NonVirtualBus=on
  Constant : Constant  Value=MessageID
  Data Type Conversion : DataTypeConversion
  Message : Outport  VectorParamsAs1DForOutWhenUnconnected=off
  wires:
  Data Type Conversion/1 -> Bus Creator1/2  "MessageStatus"
  Constant/1 -> Bus Creator1/1  "MessageID"
  State/1 -> Data Type Conversion/1
  Bus Creator1/1 -> Message/1

== system TCMSSystem/TCMSSystemPerVehicle/EnabledTCMSVehicle/OutputsPacking/TCMSDisplayOutputs/TCMSMessageEvents/DoorSystemFaults/Associated TCMS Fault ID112 ==
  State : Inport
  Bus Creator1 : BusCreator  Inputs=2  OutDataTypeStr=Bus: BD_TCMSSystem_Out_Vehicle_Display_Message  NonVirtualBus=on
  Constant : Constant  Value=MessageID
  Data Type Conversion : DataTypeConversion
  Message : Outport  VectorParamsAs1DForOutWhenUnconnected=off
  wires:
  Data Type Conversion/1 -> Bus Creator1/2  "MessageStatus"
  Constant/1 -> Bus Creator1/1  "MessageID"
  State/1 -> Data Type Conversion/1
  Bus Creator1/1 -> Message/1

== system TCMSSystem/TCMSSystemPerVehicle/EnabledTCMSVehicle/OutputsPacking/TCMSDisplayOutputs/TCMSMessageEvents/DoorSystemFaults/Associated TCMS Fault ID113 ==
  State : Inport
  Bus Creator1 : BusCreator  Inputs=2  OutDataTypeStr=Bus: BD_TCMSSystem_Out_Vehicle_Display_Message  NonVirtualBus=on
  Constant : Constant  Value=MessageID
  Data Type Conversion : DataTypeConversion
  Message : Outport  VectorParamsAs1DForOutWhenUnconnected=off
  wires:
  Data Type Conversion/1 -> Bus Creator1/2  "MessageStatus"
  Constant/1 -> Bus Creator1/1  "MessageID"
  State/1 -> Data Type Conversion/1
  Bus Creator1/1 -> Message/1

== system TCMSSystem/TCMSSystemPerVehicle/EnabledTCMSVehicle/OutputsPacking/TCMSDisplayOutputs/TCMSMessageEvents/DoorSystemFaults/Associated TCMS Fault ID114 ==
  State : Inport
  Bus Creator1 : BusCreator  Inputs=2  OutDataTypeStr=Bus: BD_TCMSSystem_Out_Vehicle_Display_Message  NonVirtualBus=on
  Constant : Constant  Value=MessageID
  Data Type Conversion : DataTypeConversion
  Message : Outport  VectorParamsAs1DForOutWhenUnconnected=off
  wires:
  Data Type Conversion/1 -> Bus Creator1/2  "MessageStatus"
  Constant/1 -> Bus Creator1/1  "MessageID"
  State/1 -> Data Type Conversion/1
  Bus Creator1/1 -> Message/1

== system TCMSSystem/TCMSSystemPerVehicle/EnabledTCMSVehicle/OutputsPacking/TCMSDisplayOutputs/TCMSMessageEvents/DoorSystemFaults/Associated TCMS Fault ID115 ==
  State : Inport
  Bus Creator1 : BusCreator  Inputs=2  OutDataTypeStr=Bus: BD_TCMSSystem_Out_Vehicle_Display_Message  NonVirtualBus=on
  Constant : Constant  Value=MessageID
  Data Type Conversion : DataTypeConversion
  Message : Outport  VectorParamsAs1DForOutWhenUnconnected=off
  wires:
  Data Type Conversion/1 -> Bus Creator1/2  "MessageStatus"
  Constant/1 -> Bus Creator1/1  "MessageID"
  State/1 -> Data Type Conversion/1
  Bus Creator1/1 -> Message/1

== system TCMSSystem/TCMSSystemPerVehicle/EnabledTCMSVehicle/OutputsPacking/TCMSDisplayOutputs/TCMSMessageEvents/DoorSystemFaults/Associated TCMS Fault ID116 ==
  State : Inport
  Bus Creator1 : BusCreator  Inputs=2  OutDataTypeStr=Bus: BD_TCMSSystem_Out_Vehicle_Display_Message  NonVirtualBus=on
  Constant : Constant  Value=MessageID
  Data Type Conversion : DataTypeConversion
  Message : Outport  VectorParamsAs1DForOutWhenUnconnected=off
  wires:
  Data Type Conversion/1 -> Bus Creator1/2  "MessageStatus"
  Constant/1 -> Bus Creator1/1  "MessageID"
  State/1 -> Data Type Conversion/1
  Bus Creator1/1 -> Message/1

== system TCMSSystem/TCMSSystemPerVehicle/EnabledTCMSVehicle/OutputsPacking/TCMSDisplayOutputs/TCMSMessageEvents/DoorSystemFaults/Associated TCMS Fault ID117 ==
  State : Inport
  Bus Creator1 : BusCreator  Inputs=2  OutDataTypeStr=Bus: BD_TCMSSystem_Out_Vehicle_Display_Message  NonVirtualBus=on
  Constant : Constant  Value=MessageID
  Data Type Conversion : DataTypeConversion
  Message : Outport  VectorParamsAs1DForOutWhenUnconnected=off
  wires:
  Data Type Conversion/1 -> Bus Creator1/2  "MessageStatus"
  Constant/1 -> Bus Creator1/1  "MessageID"
  State/1 -> Data Type Conversion/1
  Bus Creator1/1 -> Message/1

== system TCMSSystem/TCMSSystemPerVehicle/EnabledTCMSVehicle/OutputsPacking/TCMSDisplayOutputs/TCMSMessageEvents/DoorSystemFaults/Associated TCMS Fault ID118 ==
  State : Inport
  Bus Creator1 : BusCreator  Inputs=2  OutDataTypeStr=Bus: BD_TCMSSystem_Out_Vehicle_Display_Message  NonVirtualBus=on
  Constant : Constant  Value=MessageID
  Data Type Conversion : DataTypeConversion
  Message : Outport  VectorParamsAs1DForOutWhenUnconnected=off
  wires:
  Data Type Conversion/1 -> Bus Creator1/2  "MessageStatus"
  Constant/1 -> Bus Creator1/1  "MessageID"
  State/1 -> Data Type Conversion/1
  Bus Creator1/1 -> Message/1

== system TCMSSystem/TCMSSystemPerVehicle/EnabledTCMSVehicle/OutputsPacking/TCMSDisplayOutputs/TCMSMessageEvents/DoorSystemFaults/Associated TCMS Fault ID119 ==
  State : Inport
  Bus Creator1 : BusCreator  Inputs=2  OutDataTypeStr=Bus: BD_TCMSSystem_Out_Vehicle_Display_Message  NonVirtualBus=on
  Constant : Constant  Value=MessageID
  Data Type Conversion : DataTypeConversion
  Message : Outport  VectorParamsAs1DForOutWhenUnconnected=off
  wires:
  Bus Creator1/1 -> Message/1
  State/1 -> Data Type Conversion/1
  Constant/1 -> Bus Creator1/1  "MessageID"
  Data Type Conversion/1 -> Bus Creator1/2  "MessageStatus"

== system TCMSSystem/TCMSSystemPerVehicle/EnabledTCMSVehicle/OutputsPacking/TCMSDisplayOutputs/TCMSMessageEvents/DoorSystemFaults/Associated TCMS Fault ID12 ==
  State : Inport
  Bus Creator1 : BusCreator  Inputs=2  OutDataTypeStr=Bus: BD_TCMSSystem_Out_Vehicle_Display_Message  NonVirtualBus=on
  Constant : Constant  Value=MessageID
  Data Type Conversion : DataTypeConversion
  Message : Outport  VectorParamsAs1DForOutWhenUnconnected=off
  wires:
  Bus Creator1/1 -> Message/1
  State/1 -> Data Type Conversion/1
  Constant/1 -> Bus Creator1/1  "MessageID"
  Data Type Conversion/1 -> Bus Creator1/2  "MessageStatus"

== system TCMSSystem/TCMSSystemPerVehicle/EnabledTCMSVehicle/OutputsPacking/TCMSDisplayOutputs/TCMSMessageEvents/DoorSystemFaults/Associated TCMS Fault ID120 ==
  State : Inport
  Bus Creator1 : BusCreator  Inputs=2  OutDataTypeStr=Bus: BD_TCMSSystem_Out_Vehicle_Display_Message  NonVirtualBus=on
  Constant : Constant  Value=MessageID
  Data Type Conversion : DataTypeConversion
  Message : Outport  VectorParamsAs1DForOutWhenUnconnected=off
  wires:
  Bus Creator1/1 -> Message/1
  State/1 -> Data Type Conversion/1
  Constant/1 -> Bus Creator1/1  "MessageID"
  Data Type Conversion/1 -> Bus Creator1/2  "MessageStatus"
